simulink model "trustaimerge"  (R2022b)
settings: Solver=FixedStepAuto  StartTime=0.0  StopTime=inf  RelTol=1e-3
libraries: robotlib x5
settings Model: Creator=yuweiyang  LastModifiedBy=sprinkle
settings OptimizationCC: EnhancedBackFolding=on  PassReuseOutputArgsAs=Individual arguments  ZeroExternalMemoryAtStartup=off  ZeroInternalMemoryAtStartup=off  MaxStackSize=64  OptimizeBlockOrder=speed  DifferentSizesBufferReuse=on  OptimizationCustomize=off  EfficientTunableParamExpr=on
settings DebuggingCC: ParameterTunabilityLossMsg=error
settings HardwareCC: ProdBitPerPointer=32  ProdBitPerSizeT=32  ProdBitPerPtrDiffT=32  ProdLargestAtomicFloat=None  ProdIntDivRoundTo=Undefined  ProdEndianess=Unspecified  ProdWordSize=32  ProdHWDeviceType=Generic->Unspecified (assume 32-bit Generic)
settings SFSimCC: MATLABDynamicMemAlloc=off
settings RTWCC: Description=Embedded Coder  SystemTargetFile=ert.tlc  HardwareBoard=Robot Operating System (ROS)  TLCOptions="-aInlineSetEventsForThisBaseRateFcn=TLC_FALSE -aSuppressMultiTaskScheduler=TLC_FALSE  -aRateBasedStepFcn=0"  TemplateMakefile=ert_default_tmf  Toolchain=Catkin  TargetLang=C++
settings CodeAppCC: ForceParamTrailComments=on  IgnoreCustomStorageClasses=off  OperatorAnnotations=on  SimulinkDataObjDesc=on  SFDataObjDesc=on  InsertBlockDesc=on

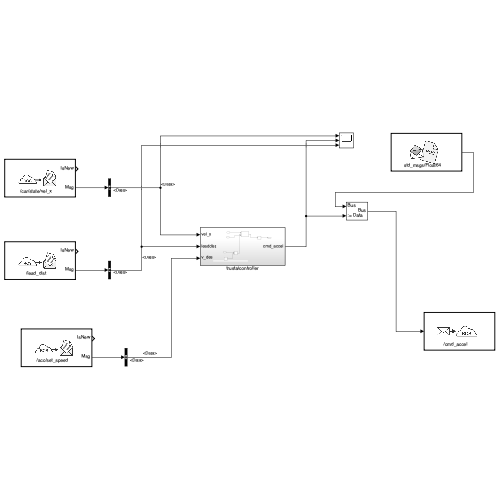
[thumbnail: Simulink's stored preview of the top-level diagram]
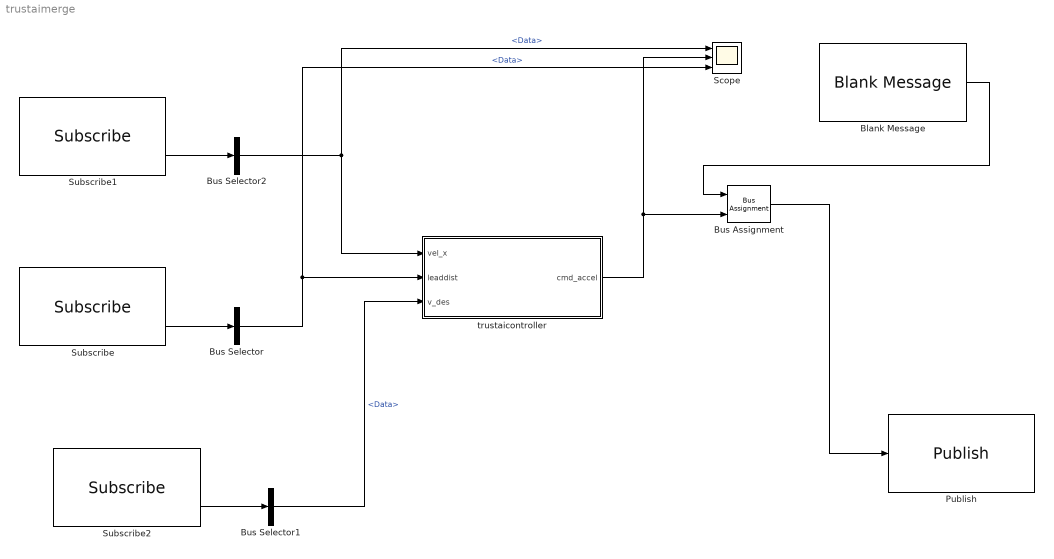
== system trustaimerge ==
  Blank Message : robotlib/Blank Message  messageClass=Message  entityType=std_msgs/Float64  messageType=std_msgs/Float64  SampleTime=inf  legacyBusStruct=off
  Bus Assignment : BusAssignment  AssignedSignals=Data
  Bus Selector : BusSelector  OutputSignals=Data
  Bus Selector1 : BusSelector  OutputSignals=Data
  Bus Selector2 : BusSelector  OutputSignals=Data
  Publish : robotlib/Publish  topicSource=Specify your own  topic=/cmd_accel  messageType=std_msgs/Float64  legacyBusStruct=off  messageQueueLength=1
  Scope : Scope  NumInputPorts=3
  Subscribe : robotlib/Subscribe  topicSource=Specify your own  topic=/lead_dist  messageType=std_msgs/Float64  SampleTime=-1  legacyBusStruct=off  messageQueueLength=1
  Subscribe1 : robotlib/Subscribe  topicSource=Specify your own  topic=/car/state/vel_x  messageType=std_msgs/Float64  SampleTime=-1  legacyBusStruct=off  messageQueueLength=1
  Subscribe2 : robotlib/Subscribe  topicSource=Specify your own  topic=/acc/set_speed  messageType=std_msgs/Float64  SampleTime=-1  legacyBusStruct=off  messageQueueLength=1
  trustaicontroller : Subsystem
  wires:
  Subscribe/2 -> Bus Selector/1
  Subscribe1/2 -> Bus Selector2/1
  Bus Assignment/1 -> Publish/1
  Bus Selector/1 -> trustaicontroller/2(leaddist), Scope/3  "<Data>"
  Bus Selector2/1 -> trustaicontroller/1(vel_x), Scope/1  "<Data>"
  Blank Message/1 -> Bus Assignment/1
  trustaicontroller/1(cmd_accel) -> Scope/2, Bus Assignment/2
  Subscribe2/2 -> Bus Selector1/1
  Bus Selector1/1 -> trustaicontroller/3(v_des)  "<Data>"

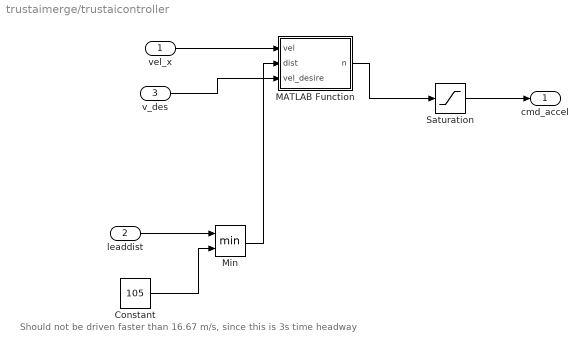
== system trustaimerge/trustaicontroller ==
  note: Should not be driven faster than 16.67 m/s, since this is 3s time headway
  vel_x : Inport
  leaddist : Inport  Port=2
  v_des : Inport  Port=3
  Constant : Constant  Value=105
  MATLAB Function : MATLAB Function  TreatAsAtomicUnit=on
  Min : MinMax  Inputs=2
  Saturation : Saturate
  cmd_accel : Outport
  wires:
  MATLAB Function/1(n) -> Saturation/1
  vel_x/1 -> MATLAB Function/1(vel)
  leaddist/1 -> Min/1
  Constant/1 -> Min/2
  Saturation/1 -> cmd_accel/1
  Min/1 -> MATLAB Function/2(dist)
  v_des/1 -> MATLAB Function/3(vel_desire)

== matlab function trustaimerge/trustaicontroller/MATLAB Function ==
  data: vel input; dist input; n output; vel_desire input
function n  = fcn(vel, dist, vel_desire)
    k1 = 0.1;
    k2 = 0.1;
    headway = 3;
%     vel_desire = 15;

    n = k1 * (dist - headway * vel) + k2 * (vel_desire - vel);
end
